simulink model "JammedActuatorAileron"  (R2018a)
settings: Solver=VariableStepAuto  StartTime=0.0  StopTime=10.0  RelTol=1e-3
libraries: simulink_extras x2
settings Model: Creator=moncayoh  LastModifiedBy=moncayoh

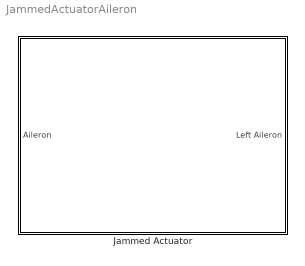
== system JammedActuatorAileron ==
  "Jammed Actuator " : Subsystem

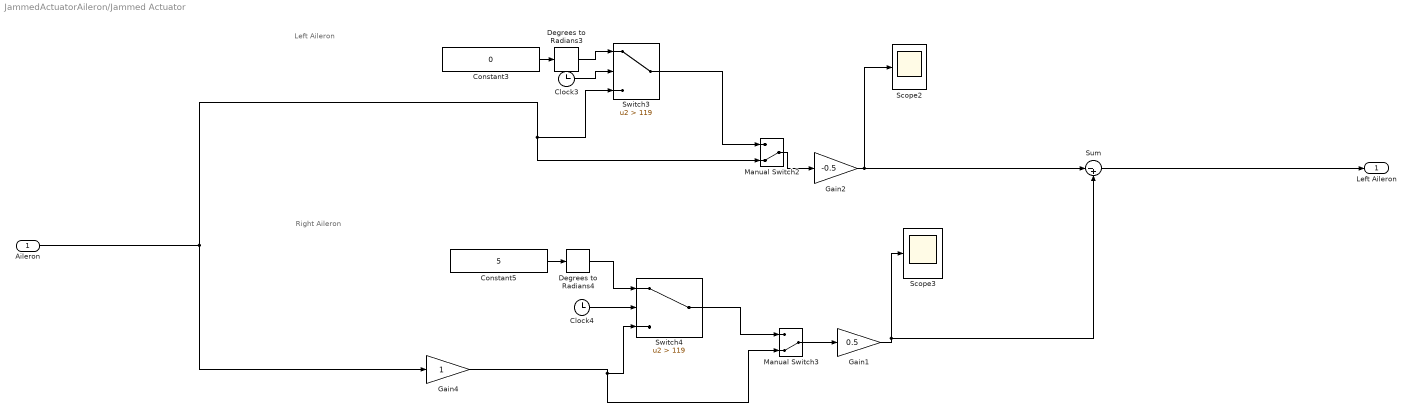
== system JammedActuatorAileron/Jammed Actuator  ==
  note: Right Aileron
  note: Left Aileron
  Aileron : Inport
  Clock3 : Clock
  Clock4 : Clock
  Constant3 : Constant  Value=0
  Constant5 : Constant  Value=5
  Degrees to Radians3 : simulink_extras/Transformations/Degrees to Radians
  Degrees to Radians4 : simulink_extras/Transformations/Degrees to Radians
  Gain1 : Gain  Gain=0.5
  Gain2 : Gain  Gain=-0.5
  Gain4 : Gain
  Manual Switch2 : ManualSwitch  CurrentSetting=0
  Manual Switch3 : ManualSwitch  CurrentSetting=0
  Scope2 : Scope
  Scope3 : Scope
  Sum : Sum  Inputs=|-+
  Switch3 : Switch  Criteria=u2 > Threshold  Threshold=119
  Switch4 : Switch  Criteria=u2 > Threshold  Threshold=119
  Left Aileron : Outport
  wires:
  Gain4/1 -> Manual Switch3/2, Switch4/3
  Aileron/1 -> Manual Switch2/2, Switch3/3, Gain4/1
  Gain1/1 -> Sum/2, Scope3/1
  Manual Switch3/1 -> Gain1/1
  Clock3/1 -> Switch3/2
  Degrees to Radians4/1 -> Switch4/1
  Gain2/1 -> Sum/1, Scope2/1
  Switch3/1 -> Manual Switch2/1
  Degrees to Radians3/1 -> Switch3/1
  Constant5/1 -> Degrees to Radians4/1
  Clock4/1 -> Switch4/2
  Switch4/1 -> Manual Switch3/1
  Manual Switch2/1 -> Gain2/1
  Constant3/1 -> Degrees to Radians3/1
  Sum/1 -> Left Aileron/1
